simulink model "Simulacao_TCC_Final"  (Simulink 9.1)
settings: Solver=VariableStepAuto  StartTime=0.0  StopTime=11000  RelTol=1e-3
undefined symbols (not defined in the file or in its folder): magnitude
libraries: sharedutil x18, vrlib x5, simulink x2, aerolibanim x1
(part 1 of 2)
settings Model: Creator=Lucas  LastModifiedBy=Lucas
settings DataIOCC: SaveFormat=Dataset
settings OptimizationCC: LifeSpan=auto
settings DebuggingCC: UnderspecifiedInitializationDetection=Simplified  MergeDetectMultiDrivingBlocksExec=error  SFUnexpectedBacktrackingDiag=error  SFNoUnconditionalDefaultTransitionDiag=error  SFExecutionAtInitializationDiag=warning
settings HardwareCC: ProdBitPerPointer=64  ProdBitPerSizeT=64  ProdBitPerPtrDiffT=64  ProdLargestAtomicFloat=Float  ProdIntDivRoundTo=Zero  ProdEndianess=LittleEndian  ProdWordSize=64  ProdHWDeviceType=Intel->x86-64 (Windows64)
settings ModelReferenceCC: PropagateSignalLabelsOutOfModel=on
settings CodeAppCC: StateflowObjectComments=off
settings GRTTargetCC: TargetLangStandard=C99 (ISO)  CombineOutputUpdateFcns=on  GRTInterface=off
settings ConfigComp: CovMetricSettings=dwe  CovHtmlReporting=off  CovSaveCumulativeToWorkspaceVar=off  CovSaveSingleToWorkspaceVar=off  CovExternalEMLEnable=on

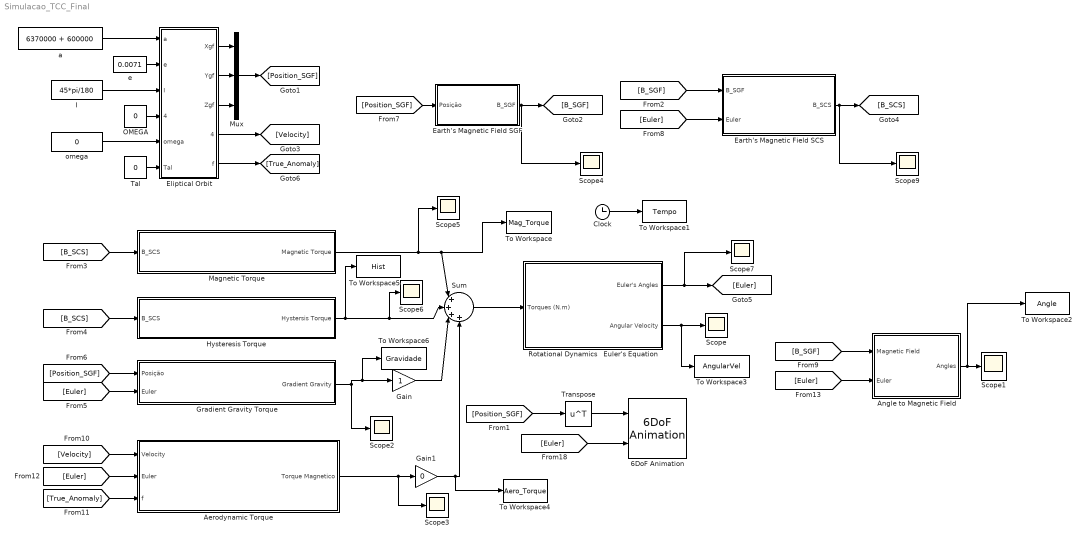
== system Simulacao_TCC_Final ==
  6DoF Animation : aerolibanim/6DoF Animation  u1=[-4000 4000 -2000 2000 -5000 -3000]  u2=10  u3=1000000*4  u4=[0 0 0]  u5=Fixed position  u6=[ 1 1 1 ] * 40000000  u7=15  u8=on
      settings: SourceProductName=Aerospace Blockset
  Aerodynamic Torque : Subsystem
  Angle to Magnetic Field : Subsystem
  Clock : Clock
  Earth's Magnetic Field SCS : Subsystem
  Earth's Magnetic Field SGF : Subsystem
  Eliptical Orbit : Subsystem
  Gain : Gain
  Gain1 : Gain  Gain=0
  Gradient Gravity Torque : Subsystem
  Hysteresis Torque : Subsystem
  I : Constant  Value=45*pi/180
  Magnetic Torque : Subsystem
  Mux : Mux  Inputs=3
  OMEGA : Constant  Value=0
  Rotational Dynamics   Euler's Equation : Subsystem
  Scope{,1..7,9} (9 alike) : Scope
  Sum : Sum  Inputs=|++++
  Tal : Constant  Value=0
  To Workspace : ToWorkspace  VariableName=Mag_Torque  SampleTime=-1
  To Workspace1 : ToWorkspace  VariableName=Tempo  SampleTime=-1
  To Workspace2 : ToWorkspace  VariableName=Angle  SampleTime=-1
  To Workspace3 : ToWorkspace  VariableName=AngularVel  SampleTime=-1
  To Workspace4 : ToWorkspace  VariableName=Aero_Torque  SampleTime=-1
  To Workspace5 : ToWorkspace  VariableName=Hist  SampleTime=-1
  To Workspace6 : ToWorkspace  VariableName=Gravidade  SampleTime=-1
  Transpose : Math  Operator=transpose  SaturateOnIntegerOverflow=on
  a : Constant  Value=6370000 + 600000
  e : Constant  Value=0.0071
  omega : Constant  Value=0
  wires:
  a/1 -> Eliptical Orbit/1(a)
  Eliptical Orbit/2(Ygf) -> Mux/2
  I/1 -> Eliptical Orbit/3(I)
  Tal/1 -> Eliptical Orbit/6(Tal)
  omega/1 -> Eliptical Orbit/5(omega)
  Eliptical Orbit/3(Zgf) -> Mux/3
  Eliptical Orbit/1(Xgf) -> Mux/1
  e/1 -> Eliptical Orbit/2(e)
  Mux/1 -> [Position_SGF]
  OMEGA/1 -> Eliptical Orbit/4(OMEGA)
  [Position_SGF] -> Earth's Magnetic Field SGF/1(Posição)
  Earth's Magnetic Field SGF/1(B_SGF) -> Scope4/1, [B_SGF]
  [B_SCS] -> Magnetic Torque/1(B_SCS)
  [B_SCS] -> Hysteresis Torque/1(B_SCS)
  [Euler] -> Gradient Gravity Torque/2(Euler)
  [Position_SGF] -> Gradient Gravity Torque/1(Posição)
  Sum/1 -> Rotational Dynamics   Euler's Equation/1(Torques (N.m))
  Magnetic Torque/1(Magnetic Torque) -> Scope5/1, To Workspace/1, Sum/1
  Hysteresis Torque/1(Hystersis Torque) -> Scope6/1, Sum/2, To Workspace5/1
  Rotational Dynamics   Euler's Equation/1(Euler's Angles) -> [Euler], Scope7/1
  [B_SGF] -> Angle to Magnetic Field/1(Magnetic Field)
  [Euler] -> Angle to Magnetic Field/2(Euler)
  Rotational Dynamics   Euler's Equation/2(Angular Velocity) -> To Workspace3/1, Scope/1
  Gradient Gravity Torque/1(Gradient Gravity) -> To Workspace6/1, Gain/1, Scope2/1
  Gain/1 -> Sum/3
  Earth's Magnetic Field SCS/1(B_SCS) -> Scope9/1, [B_SCS]
  [Euler] -> Earth's Magnetic Field SCS/2(Euler)
  [B_SGF] -> Earth's Magnetic Field SCS/1(B_SGF)
  [Euler] -> 6DoF Animation/2
  Transpose/1 -> 6DoF Animation/1
  [Position_SGF] -> Transpose/1
  Eliptical Orbit/4(Velocity) -> [Velocity]
  Eliptical Orbit/5(f) -> [True_Anomaly]
  Clock/1 -> To Workspace1/1
  Angle to Magnetic Field/1(Angles) -> To Workspace2/1, Scope1/1
  [Euler] -> Aerodynamic Torque/2(Euler)
  [True_Anomaly] -> Aerodynamic Torque/3(f)
  Aerodynamic Torque/1(Torque Magnetico) -> Scope3/1, Gain1/1
  Gain1/1 -> Sum/4, To Workspace4/1
  [Velocity] -> Aerodynamic Torque/1(Velocity)

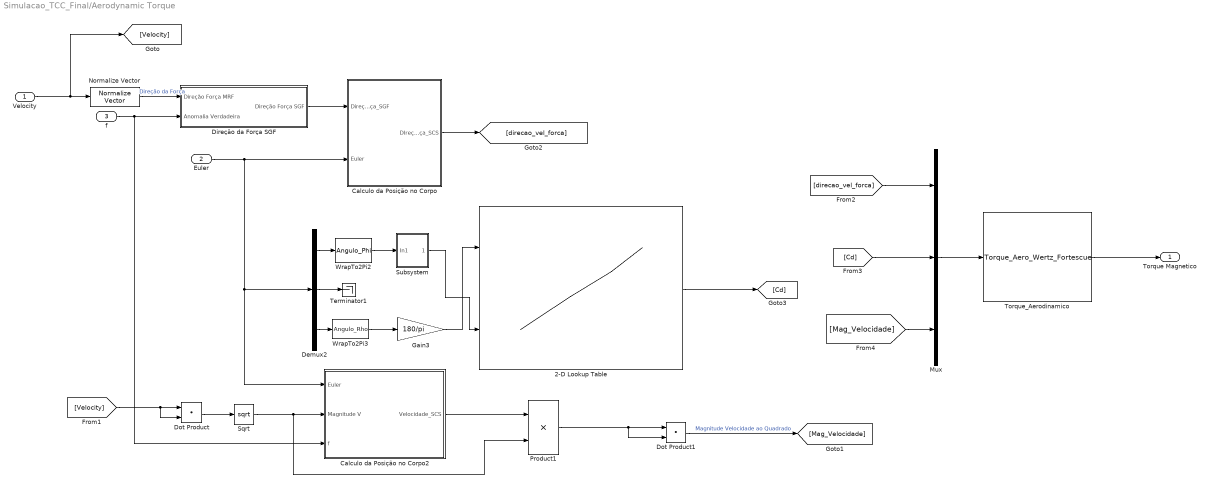
== system Simulacao_TCC_Final/Aerodynamic Torque ==
  Velocity : Inport
  Euler : Inport  Port=2
  f : Inport  Port=3
  2-D Lookup Table : Lookup_n-D  BreakpointsForDimension1=[0,45,90,135,180,225,270,315,360]  BreakpointsForDimension2=[0,10,20,30,40,50,60,70,80,90]  Table=reshape([2.7,1.93,2.7,1.93,2.7,1.93,2.7,1.93,2.47,2.7,1.9,2.47,1.9,2.7,1.9,2.47,1.9,2.45,2.7,1.85,2.25,1.85,2.7,1.85,2.25,1.85,2.43,2.7,1.83,2.07,1.83,2.7,1.83,2.07,1.83,2.41,2.7,1.8,1.95,1.8,2.7,1.8,1.95,1.8,2.39,2.7,1.8,1.95,1.8,2.7,1.8,1.95,1.8,2.39,2.7,1.83,2.07,1.83,2.7,1.83,2.07,1.83,2.41,2.7,1.85,2.25,1.85,2.7,1.85,2.25,1.85,2.43,2.7,1.9,2.47,1.9,2.7,1.9,2.47,1.9,2.47,2.7,1.93,2.7,1.93,2.7,1.93,2.7,1.93,2.47],9,10)  InternalRulePriority=Speed  RndMeth=Simplest  InputSameDT=on
  Calculo da Posição no Corpo : Subsystem
  Calculo da Posição no Corpo2 : Subsystem
  Demux2 : Demux  Outputs=3
  Direção da Força SGF : Subsystem
  Dot Product : DotProduct  InputSameDT=on  OutDataTypeStr=Inherit: Inherit via internal rule
  Dot Product1 : DotProduct  InputSameDT=on  OutDataTypeStr=Inherit: Inherit via internal rule
  Gain3 : Gain  Gain=180/pi
  Mux : Mux  Inputs=3
  Normalize Vector : vrlib/Utilities/Normalize Vector  maxzero=0
      settings: SourceProductName=Simulink 3D Animation  SourceProductBaseCode=VR
  Product1 : Product
  Sqrt : Sqrt  SaturateOnIntegerOverflow=on
  Subsystem : Subsystem
  Terminator1 : Terminator
  "Torque_Aerodinamico " : MATLABFcn  MATLABFcn=Torque_Aero_Wertz_Fortescue  OutputDimensions=3
  WrapTo2Pi2 : MATLABFcn  MATLABFcn=Angulo_Phi
  WrapTo2Pi3 : MATLABFcn  MATLABFcn=Angulo_Rho
  Torque Magnetico : Outport
  wires:
  Normalize Vector/1 -> Direção da Força SGF/1(Direção Força MRF)  "Direção da Força"
  Direção da Força SGF/1(Direção Força SGF) -> Calculo da Posição no Corpo/1(Direção_Força_SGF)
  Calculo da Posição no Corpo/1(DIreção_Força_SCS) -> [direcao_vel_forca]
  Velocity/1 -> [Velocity], Normalize Vector/1
  f/1 -> Calculo da Posição no Corpo2/3(f), Direção da Força SGF/2(Anomalia Verdadeira)
  Calculo da Posição no Corpo2/1("Velocidade_SCS ") -> Product1/1
  Dot Product/1 -> Sqrt/1
  [Velocity] -> Dot Product/2, Dot Product/1
  Euler/1 -> Demux2/1, Calculo da Posição no Corpo2/1(Euler), Calculo da Posição no Corpo/2(Euler)
  Dot Product1/1 -> [Mag_Velocidade]  "Magnitude Velocidade ao Quadrado"
  [direcao_vel_forca] -> Mux/1
  [Cd] -> Mux/2
  [Mag_Velocidade] -> Mux/3
  Mux/1 -> "Torque_Aerodinamico "/1
  "Torque_Aerodinamico "/1 -> Torque Magnetico/1
  Sqrt/1 -> Product1/2, Calculo da Posição no Corpo2/2(Magnitude V)
  Product1/1 -> Dot Product1/2, Dot Product1/1
  Demux2/2 -> Terminator1/1
  Subsystem/1(Out1) -> 2-D Lookup Table/2
  WrapTo2Pi2/1 -> Subsystem/1(In1)
  2-D Lookup Table/1 -> [Cd]
  Demux2/3 -> WrapTo2Pi3/1
  Gain3/1 -> 2-D Lookup Table/1
  Demux2/1 -> WrapTo2Pi2/1
  WrapTo2Pi3/1 -> Gain3/1

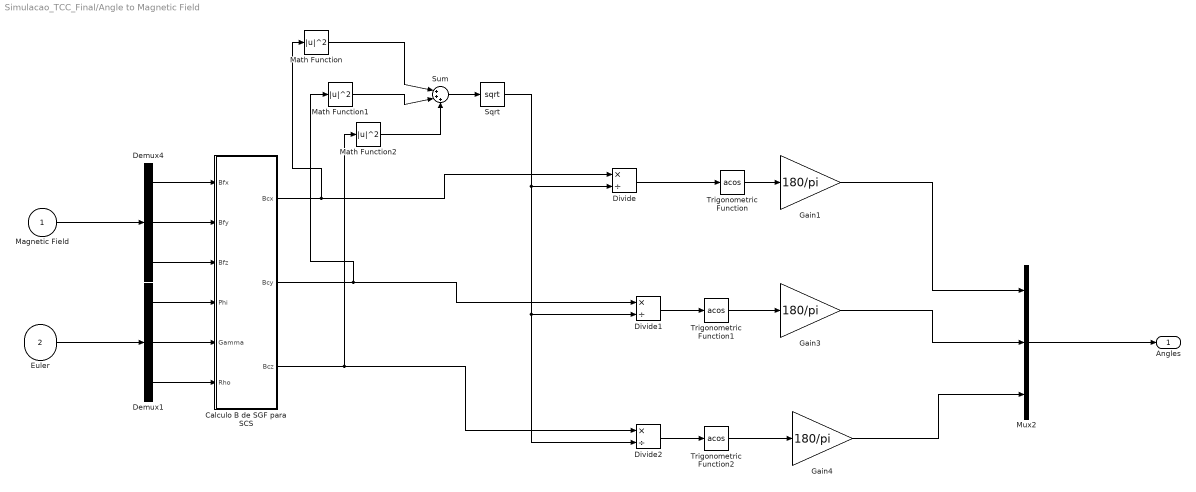
== system Simulacao_TCC_Final/Angle to Magnetic Field ==
  Magnetic Field : Inport
  Euler : Inport  Port=2
  Calculo B de SGF para SCS : Subsystem
  Demux1 : Demux  Outputs=3
  Demux4 : Demux  Outputs=3
  Divide : Product  Inputs=*/
  Divide1 : Product  Inputs=*/
  Divide2 : Product  Inputs=*/
  Gain1 : Gain  Gain=180/pi
  Gain3 : Gain  Gain=180/pi
  Gain4 : Gain  Gain=180/pi
  Math Function : Math  Operator=magnitude^2  SaturateOnIntegerOverflow=on
  Math Function1 : Math  Operator=magnitude^2  SaturateOnIntegerOverflow=on
  Math Function2 : Math  Operator=magnitude^2  SaturateOnIntegerOverflow=on
  Mux2 : Mux  Inputs=3
  Sqrt : Sqrt  SaturateOnIntegerOverflow=on
  Sum : Sum  Inputs=|+++
  Trigonometric Function : Trigonometry  Operator=acos
  Trigonometric Function1 : Trigonometry  Operator=acos
  Trigonometric Function2 : Trigonometry  Operator=acos
  Angles : Outport
  wires:
  Demux4/1 -> Calculo B de SGF para SCS/1(Bfx)
  Demux4/2 -> Calculo B de SGF para SCS/2(Bfy)
  Demux4/3 -> Calculo B de SGF para SCS/3(Bfz)
  Magnetic Field/1 -> Demux4/1
  Demux1/1 -> Calculo B de SGF para SCS/4(Phi)
  Demux1/2 -> Calculo B de SGF para SCS/5(Gamma)
  Demux1/3 -> Calculo B de SGF para SCS/6(Rho)
  Euler/1 -> Demux1/1
  Mux2/1 -> Angles/1
  Trigonometric Function2/1 -> Gain4/1
  Trigonometric Function1/1 -> Gain3/1
  Divide1/1 -> Trigonometric Function1/1
  Divide2/1 -> Trigonometric Function2/1
  Trigonometric Function/1 -> Gain1/1
  Divide/1 -> Trigonometric Function/1
  Calculo B de SGF para SCS/1(Bcx) -> Math Function/1, Divide/1
  Sqrt/1 -> Divide2/2, Divide1/2, Divide/2
  Calculo B de SGF para SCS/2(Bcy) -> Math Function1/1, Divide1/1
  Calculo B de SGF para SCS/3(Bcz) -> Divide2/1, Math Function2/1
  Gain1/1 -> Mux2/1
  Gain3/1 -> Mux2/2
  Gain4/1 -> Mux2/3
  Sum/1 -> Sqrt/1
  Math Function/1 -> Sum/1
  Math Function1/1 -> Sum/2
  Math Function2/1 -> Sum/3

== system Simulacao_TCC_Final/Earth's Magnetic Field SCS ==
  B_SGF : Inport
  Euler : Inport  Port=2
  Demux2 : Demux  Outputs=3
  Matrix Multiply : Product  Multiplication=Matrix(*)
  Matrix Multiply1 : Product  Multiplication=Matrix(*)
  Matrix Multiply2 : Product  Multiplication=Matrix(*)
  Matrix de Rotação em X : Subsystem
  Matrix de Rotação em Y : Subsystem
  Matrix de Rotação em Z : Subsystem
  B_SCS : Outport
  wires:
  Euler/1 -> Demux2/1
  Matrix Multiply/1 -> B_SCS/1
  B_SGF/1 -> Matrix Multiply/2
  Demux2/1 -> Matrix de Rotação em X/1(Phi)
  Demux2/2 -> Matrix de Rotação em Y/1(Gamma)
  Demux2/3 -> Matrix de Rotação em Z/1(Phi)
  Matrix de Rotação em X/1(Matrix Rotação  em X) -> Matrix Multiply1/1
  Matrix de Rotação em Y/1(Matrix Rotação  em Y) -> Matrix Multiply1/2
  Matrix Multiply1/1 -> Matrix Multiply2/1
  Matrix de Rotação em Z/1(Matrix Rotação  em Z) -> Matrix Multiply2/2
  Matrix Multiply2/1 -> Matrix Multiply/1

== system Simulacao_TCC_Final/Earth's Magnetic Field SGF ==
  Posição : Inport
  1 : Math  Operator=magnitude^2  SaturateOnIntegerOverflow=on
  2 : Math  Operator=magnitude^2  SaturateOnIntegerOverflow=on
  3 : Math  Operator=magnitude^2  SaturateOnIntegerOverflow=on
  Calculo Campo Magnetico LATITUDE : Subsystem
  Demux : Demux  Outputs=3
  Demux1 : Demux  Outputs=3
  Mux2 : Mux  Inputs=3
  Raio Terra : Constant  Value=6370000
  SGF para SGG : Subsystem
  SGF para SGG1 : Subsystem
  SGF para SGG2 : Subsystem
  SGF para SGG3 : Subsystem
  Sist Esferico - > SMG1 : Subsystem
  Sqrt : Sqrt  SaturateOnIntegerOverflow=on
  Sum : Sum  Inputs=|+++
  B_SGF : Outport
  wires:
  Demux/1 -> 1/1
  Demux/2 -> 2/1
  Raio Terra/1 -> Calculo Campo Magnetico LATITUDE/2(Raio Terra)
  Sum/1 -> Sqrt/1
  1/1 -> Sum/1
  2/1 -> Sum/2
  3/1 -> Sum/3
  Demux/3 -> 3/1
  Posição/1 -> SGF para SGG/1(Posição_SGF), Demux/1
  Sqrt/1 -> [Raio]  "RAIO"
  SGF para SGG/1(Posição_SGG) -> SGF para SGG1/1(Posição_SGG)
  SGF para SGG1/1(Posição_SMG) -> Demux1/1
  Demux1/3 -> Calculo Campo Magnetico LATITUDE/1(Zgm), Sist Esferico - > SMG1/6(Zm)
  [Raio] -> Calculo Campo Magnetico LATITUDE/3(Raio)
  Calculo Campo Magnetico LATITUDE/1(Br) -> Sist Esferico - > SMG1/1(Br)
  Calculo Campo Magnetico LATITUDE/2(Btheta) -> Sist Esferico - > SMG1/2(Btheta)
  Calculo Campo Magnetico LATITUDE/3(Delta) -> Sist Esferico - > SMG1/3(Delta)
  Demux1/1 -> Sist Esferico - > SMG1/4(Xm)
  Demux1/2 -> Sist Esferico - > SMG1/5(Ym)
  Mux2/1 -> SGF para SGG2/1(B_SMG)
  Sist Esferico - > SMG1/1(Bmx) -> Mux2/1
  Sist Esferico - > SMG1/2(Bmy) -> Mux2/2
  Sist Esferico - > SMG1/3(Bmz) -> Mux2/3
  SGF para SGG2/1(B_SGG) -> SGF para SGG3/1(B_SGG)
  SGF para SGG3/1(B_SGF) -> B_SGF/1

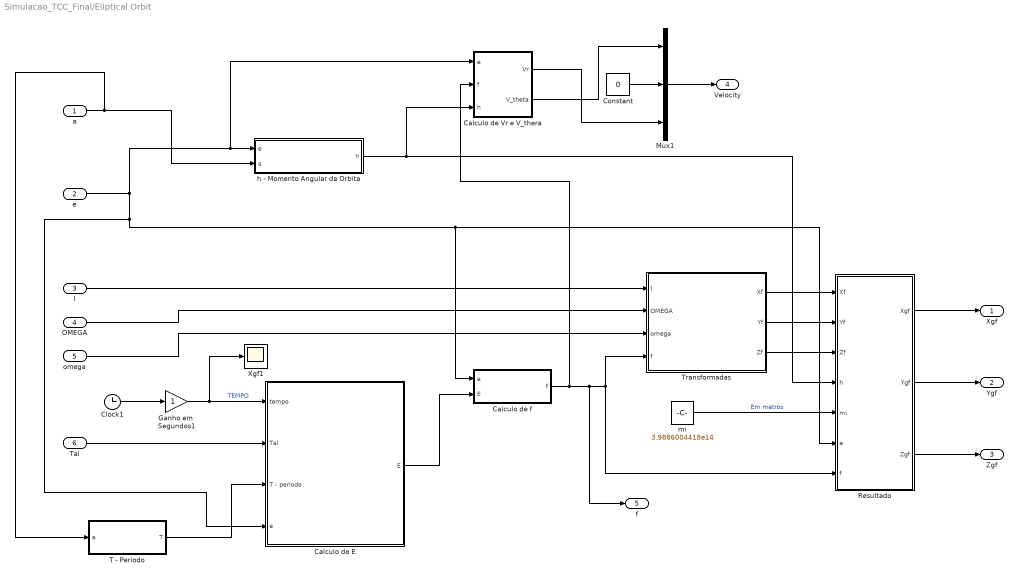
== system Simulacao_TCC_Final/Eliptical Orbit ==
  a : Inport
  e : Inport  Port=2
  I : Inport  Port=3
  OMEGA : Inport  Port=4
  omega : Inport  Port=5
  Tal : Inport  Port=6
  Calculo de E : Subsystem
  Calculo de Vr e V_thera : Subsystem
  Calculo de f : Subsystem
  Clock1 : Clock
  Constant : Constant  Value=0
  Ganho em  Segundos1 : Gain
  Mux1 : Mux  Inputs=3
  Resultado : Subsystem
  T - Periodo : Subsystem
  Transformadas : Subsystem
  Xgf1 : Scope
  h - Momento Angular da Orbita : Subsystem
  mi : Constant  Value=3.9886004418e14
  Xgf : Outport
  Ygf : Outport  Port=2
  Zgf : Outport  Port=3
  Velocity : Outport  Port=4
  f : Outport  Port=5
  wires:
  Transformadas/2(Yf) -> Resultado/2(Yf)
  Transformadas/3(Zf) -> Resultado/3(Zf)
  Calculo de f/1(f) -> Calculo de Vr e V_thera/2(f), f/1, Transformadas/4(f), Resultado/7(f)
  Transformadas/1(Xf) -> Resultado/1(Xf)
  mi/1 -> Resultado/5(mi)  "Em metros"
  e/1 -> Calculo de E/4("e  "), Calculo de f/1(e), Resultado/6(e), Calculo de Vr e V_thera/1(e), h - Momento Angular da Orbita/1(e)
  h - Momento Angular da Orbita/1(h) -> Calculo de Vr e V_thera/3(h), Resultado/4(h)
  I/1 -> Transformadas/1(I)
  OMEGA/1 -> Transformadas/2(OMEGA)
  omega/1 -> Transformadas/3(omega)
  Resultado/3(Zgf) -> Zgf/1
  Resultado/2(Ygf) -> Ygf/1
  Resultado/1(Xgf) -> Xgf/1
  Tal/1 -> Calculo de E/2(Tal)
  T - Periodo/1(T) -> Calculo de E/3(T - periodo)
  a/1 -> T - Periodo/1(a), h - Momento Angular da Orbita/2(a)
  Clock1/1 -> Ganho em  Segundos1/1
  Ganho em  Segundos1/1 -> Xgf1/1, Calculo de E/1(tempo)  "TEMPO"
  Calculo de E/1(E) -> Calculo de f/2(E)
  Calculo de Vr e V_thera/1(Vr) -> Mux1/3
  Constant/1 -> Mux1/2
  Calculo de Vr e V_thera/2(V_theta) -> Mux1/1
  Mux1/1 -> Velocity/1

== system Simulacao_TCC_Final/Gradient Gravity Torque ==
  note: Vetor Nadir
  Posição : Inport
  Euler : Inport  Port=2
  3u. : Gain  Gain=3*(3.9886004418e14)
  Calculo da Posição no Corpo : Subsystem
  Constant : Constant  Value=0
  Cross Product : vrlib/Utilities/Cross Product
      settings: SourceProductBaseCode=VR
  Divide : Product  Inputs=*/
  Dot Product : DotProduct  InputSameDT=on  OutDataTypeStr=Inherit: Inherit via internal rule
  Gain : Gain  Gain=-1
  Gain1 : Gain  Gain=-1
  Ixx : Constant  Value=0.00182
  Iyy : Constant  Value=0.00185
  Izz : Constant  Value=0.00220
  Math Function : Math  Operator=square  SaturateOnIntegerOverflow=on
  Matrix Multiply : Product  Multiplication=Matrix(*)
  Matriz de Inercia : sharedutil/Create 3x3 Matrix  aMode=aMode
  Normalize Vector : vrlib/Utilities/Normalize Vector  maxzero=0
      settings: SourceProductName=Simulink 3D Animation  SourceProductBaseCode=VR
  Gradient Gravity : Outport
  wires:
  Euler/1 -> Calculo da Posição no Corpo/2(Euler)
  Calculo da Posição no Corpo/1(X_SCS) -> Gain1/1, Normalize Vector/1
  Normalize Vector/1 -> Gain/1
  Gain/1 -> Matrix Multiply/2
  Posição/1 -> Dot Product/2, Dot Product/1, Calculo da Posição no Corpo/1(X_SGF)
  Constant/1 -> Matriz de Inercia/4, Matriz de Inercia/3, Matriz de Inercia/2, Matriz de Inercia/6, Matriz de Inercia/7, Matriz de Inercia/8
  Ixx/1 -> Matriz de Inercia/1
  Iyy/1 -> Matriz de Inercia/5
  Izz/1 -> Matriz de Inercia/9
  Matriz de Inercia/1 -> Matrix Multiply/1
  Divide/1 -> Cross Product/1
  Matrix Multiply/1 -> Cross Product/2
  Cross Product/1 -> Gradient Gravity/1
  Dot Product/1 -> Math Function/1
  Math Function/1 -> Divide/2
  3u./1 -> Divide/1
  Gain1/1 -> 3u./1

== system Simulacao_TCC_Final/Hysteresis Torque ==
  B_SCS : Inport
  1/mu : Gain  Gain=1/(1.256637061435917e-06)
  1/mu. : Constant  Value=1/(1.256637061435917e-06)
  Cross Product : vrlib/Utilities/Cross Product
      settings: SourceProductBaseCode=VR
  Hysteresys : Subsystem
  V/mu : Product  RndMeth=Zero
  Volume Material : Constant  Value=[5e-9 7e-08 7e-08]
  m : Product  RndMeth=Zero
  Hystersis Torque : Outport
  wires:
  B_SCS/1 -> 1/mu/1, Cross Product/2
  m/1 -> Cross Product/1
  Hysteresys/1(B) -> m/1
  1/mu/1 -> Hysteresys/1(H)
  Cross Product/1 -> Hystersis Torque/1
  Volume Material/1 -> V/mu/1
  1/mu./1 -> V/mu/2
  V/mu/1 -> m/2

== system Simulacao_TCC_Final/Magnetic Torque ==
  note: T = m X B
  B_SCS : Inport
  Cross Product : vrlib/Utilities/Cross Product
      settings: SourceProductBaseCode=VR
  Imãs : Constant  Value=[0.7 0 0]
  Magnetic Torque : Outport
  wires:
  B_SCS/1 -> Cross Product/2  "Magnetic Field on Body"
  Imãs/1 -> Cross Product/1
  Cross Product/1 -> Magnetic Torque/1

== system Simulacao_TCC_Final/Rotational Dynamics   Euler's Equation ==
  Torques (N.m) : Inport
  Euler Angles : Subsystem
  Euler's Equation Body - Framed : Subsystem
  Euler's Angles : Outport
  Angular Velocity : Outport  Port=2
  wires:
  Torques (N.m)/1 -> Euler's Equation Body - Framed/1(Torques)
  Euler's Equation Body - Framed/1(Angular Velocity Body Frame) -> Angular Velocity/1, Euler Angles/1(Angular Velocity Body Frame)
  Euler Angles/1(Euler's Angle) -> Euler's Angles/1

== system Simulacao_TCC_Final/Aerodynamic Torque/Calculo da Posição no Corpo ==
  Direção_Força_SGF : Inport
  Euler : Inport  Port=2
  Demux1 : Demux  Outputs=3
  Matrix Multiply : Product  Multiplication=Matrix(*)
  Matrix Multiply1 : Product  Multiplication=Matrix(*)
  Matrix Multiply2 : Product  Multiplication=Matrix(*)
  Matrix de Rotação em X : Subsystem
  Matrix de Rotação em Y : Subsystem
  Matrix de Rotação em Z : Subsystem
  DIreção_Força_SCS : Outport
  wires:
  Direção_Força_SGF/1 -> Matrix Multiply/2
  Matrix Multiply/1 -> DIreção_Força_SCS/1
  Matrix de Rotação em X/1(Matrix Rotação  em X) -> Matrix Multiply1/1
  Euler/1 -> Demux1/1
  Demux1/3 -> Matrix de Rotação em Z/1(Phi)
  Matrix de Rotação em Z/1(Matrix Rotação  em Z) -> Matrix Multiply2/2
  Matrix de Rotação em Y/1(Matrix Rotação  em Y) -> Matrix Multiply1/2
  Demux1/2 -> Matrix de Rotação em Y/1(Gamma)
  Matrix Multiply1/1 -> Matrix Multiply2/1
  Matrix Multiply2/1 -> Matrix Multiply/1
  Demux1/1 -> Matrix de Rotação em X/1(Phi)

== system Simulacao_TCC_Final/Aerodynamic Torque/Calculo da Posição no Corpo2 ==
  Euler : Inport
  Magnitude V : Inport  Port=2
  f : Inport  Port=3
  Constant : Constant  Value=-1
  Constant1 : Constant  Value=6370000 + 300000
  Constant2 : Constant  Value=0
  Constant3 : Constant  Value=7.27e-5
  Demux1 : Demux  Outputs=3
  Divide : Product  Inputs=*/
  Matrix Multiply : Product  Multiplication=Matrix(*)
  Matrix Multiply1 : Product  Multiplication=Matrix(*)
  Matrix Multiply2 : Product  Multiplication=Matrix(*)
  Matrix de Rotação em X : Subsystem
  Matrix de Rotação em Y : Subsystem
  Matrix de Rotação em Z : Subsystem
  Mux : Mux  Inputs=3
  Product : Product  Inputs=3
  Trigonometric Function : Trigonometry  Operator=cos
  "Velocidade_SCS " : Outport
  wires:
  Matrix Multiply/1 -> "Velocidade_SCS "/1
  Matrix de Rotação em X/1(Matrix Rotação  em X) -> Matrix Multiply1/1
  Euler/1 -> Demux1/1
  Demux1/3 -> Matrix de Rotação em Z/1(Phi)
  Matrix de Rotação em Z/1(Matrix Rotação  em Z) -> Matrix Multiply2/2
  Matrix de Rotação em Y/1(Matrix Rotação  em Y) -> Matrix Multiply1/2
  Demux1/2 -> Matrix de Rotação em Y/1(Gamma)
  Matrix Multiply1/1 -> Matrix Multiply2/1
  Matrix Multiply2/1 -> Matrix Multiply/1
  Demux1/1 -> Matrix de Rotação em X/1(Phi)
  Mux/1 -> Matrix Multiply/2
  Constant/1 -> Mux/1
  Divide/1 -> Product/2
  Magnitude V/1 -> Divide/2
  Constant1/1 -> Divide/1
  f/1 -> Trigonometric Function/1
  Trigonometric Function/1 -> Product/1
  Constant2/1 -> Mux/3
  Product/1 -> Mux/2
  Constant3/1 -> Product/3

== system Simulacao_TCC_Final/Aerodynamic Torque/Direção da Força SGF ==
  Direção Força MRF : Inport
  Anomalia Verdadeira : Inport  Port=2
  Add : Sum
  Constant : Constant  Value=pi/2
  Constant1 : Constant  Value=0
  Demux : Demux  Outputs=3
  Mux1 : Mux  Inputs=3
  Product : Product
  Product1 : Product
  Terminator1 : Terminator
  Terminator2 : Terminator
  Trigonometric Function : Trigonometry  Operator=cos
  Trigonometric Function1 : Trigonometry
  Direção Força SGF : Outport
  wires:
  Mux1/1 -> Direção Força SGF/1
  Constant/1 -> Add/1
  Anomalia Verdadeira/1 -> Add/2
  Add/1 -> Trigonometric Function1/1, Trigonometric Function/1
  Direção Força MRF/1 -> Demux/1
  Product1/1 -> Mux1/2
  Trigonometric Function/1 -> Product/1
  Trigonometric Function1/1 -> Product1/1
  Demux/1 -> Product1/2, Product/2
  Product/1 -> Mux1/1
  Constant1/1 -> Mux1/3
  Demux/3 -> Terminator2/1
  Demux/2 -> Terminator1/1

== system Simulacao_TCC_Final/Aerodynamic Torque/Subsystem ==
  In1 : Inport
  Gain1 : Gain  Gain=180/pi
  If : If  IfExpression=u1 > 90
  If Action Subsystem1 : Subsystem  TreatAsAtomicUnit=on
  If Action Subsystem2 : Subsystem  TreatAsAtomicUnit=on
  Merge : Merge
  Out1 : Outport
  wires:
  In1/1 -> Gain1/1
  Gain1/1 -> [A], If/1
  Merge/1 -> Out1/1
  If/1 -> If Action Subsystem1/Action
  [A] -> If Action Subsystem1/1(In1)
  If/2 -> If Action Subsystem2/Action
  [A] -> If Action Subsystem2/1(In1)
  If Action Subsystem2/1(Out1) -> Merge/2
  If Action Subsystem1/1(Out1) -> Merge/1

== system Simulacao_TCC_Final/Angle to Magnetic Field/Calculo B de SGF para SCS ==
  Bfx : Inport
  Bfy : Inport  Port=2
  Bfz : Inport  Port=3
  Phi : Inport  Port=4
  Gamma : Inport  Port=5
  Rho : Inport  Port=6
  "Calculo de X " : Subsystem
  Calculo de Y : Subsystem
  Calculo de Z : Subsystem
  Gain : Gain
  Bcx : Outport
  Bcy : Outport  Port=2
  Bcz : Outport  Port=3
  wires:
  Bfz/1 -> Calculo de Z/3(Bfz), Calculo de Y/3(Bfz), "Calculo de X "/3(Bfz)
  "Calculo de X "/1(X) -> Gain/1
  Calculo de Y/1(Y) -> Bcy/1
  Calculo de Z/1(Z) -> Bcz/1
  Bfx/1 -> Calculo de Z/1(Bfx), Calculo de Y/1(Bfx), "Calculo de X "/1(Bfx)
  Bfy/1 -> Calculo de Z/2(Bfy), Calculo de Y/2(Bfy), "Calculo de X "/2(Bfy)
  Phi/1 -> Calculo de Z/4(Phi), Calculo de Y/4(Phi)
  Gamma/1 -> "Calculo de X "/4(Gamma), Calculo de Z/5(Gamma), Calculo de Y/5(Gamma)
  Rho/1 -> "Calculo de X "/5(Rho), Calculo de Z/6(Rho), Calculo de Y/6(Rho)
  Gain/1 -> Bcx/1

== system Simulacao_TCC_Final/Earth's Magnetic Field SCS/Matrix de Rotação em X ==
  Phi : Inport
  Constant : Constant
  Constant{1..4} (4 alike) : Constant  Value=0
  Create 3x3 Matrix : sharedutil/Create 3x3 Matrix  aMode=aMode
  Gain : Gain  Gain=-1
  Trigonometric Function : Trigonometry
  Trigonometric Function1 : Trigonometry  Operator=cos
  Trigonometric Function2 : Trigonometry
  Trigonometric Function3 : Trigonometry  Operator=cos
  Matrix Rotação  em X : Outport
  wires:
  Constant/1 -> Create 3x3 Matrix/1
  Constant1/1 -> Create 3x3 Matrix/2
  Constant2/1 -> Create 3x3 Matrix/3
  Constant3/1 -> Create 3x3 Matrix/4
  Trigonometric Function1/1 -> Create 3x3 Matrix/5
  Trigonometric Function/1 -> Create 3x3 Matrix/6
  Constant4/1 -> Create 3x3 Matrix/7
  Phi/1 -> Trigonometric Function2/1, Trigonometric Function3/1, Trigonometric Function/1, Trigonometric Function1/1
  Trigonometric Function2/1 -> Gain/1
  Gain/1 -> Create 3x3 Matrix/8
  Trigonometric Function3/1 -> Create 3x3 Matrix/9
  Create 3x3 Matrix/1 -> Matrix Rotação  em X/1

== system Simulacao_TCC_Final/Earth's Magnetic Field SCS/Matrix de Rotação em Y ==
  Gamma : Inport
  Constant : Constant
  Constant{1..4} (4 alike) : Constant  Value=0
  Create 3x3 Matrix : sharedutil/Create 3x3 Matrix  aMode=aMode
  Gain : Gain  Gain=-1
  Trigonometric Function : Trigonometry
  Trigonometric Function1 : Trigonometry  Operator=cos
  Trigonometric Function2 : Trigonometry
  Trigonometric Function3 : Trigonometry  Operator=cos
  Matrix Rotação  em Y : Outport
  wires:
  Create 3x3 Matrix/1 -> Matrix Rotação  em Y/1
  Trigonometric Function1/1 -> Create 3x3 Matrix/1
  Trigonometric Function2/1 -> Gain/1
  Constant1/1 -> Create 3x3 Matrix/2
  Gain/1 -> Create 3x3 Matrix/3
  Constant2/1 -> Create 3x3 Matrix/4
  Constant/1 -> Create 3x3 Matrix/5
  Constant3/1 -> Create 3x3 Matrix/6
  Trigonometric Function/1 -> Create 3x3 Matrix/7
  Constant4/1 -> Create 3x3 Matrix/8
  Trigonometric Function3/1 -> Create 3x3 Matrix/9
  Gamma/1 -> Trigonometric Function/1, Trigonometric Function3/1, Trigonometric Function1/1, Trigonometric Function2/1

== system Simulacao_TCC_Final/Earth's Magnetic Field SCS/Matrix de Rotação em Z ==
  Phi : Inport
  Constant : Constant
  Constant{1..4} (4 alike) : Constant  Value=0
  Create 3x3 Matrix : sharedutil/Create 3x3 Matrix  aMode=aMode
  Gain : Gain  Gain=-1
  Trigonometric Function : Trigonometry
  Trigonometric Function1 : Trigonometry  Operator=cos
  Trigonometric Function2 : Trigonometry
  Trigonometric Function3 : Trigonometry  Operator=cos
  Matrix Rotação  em Z : Outport
  wires:
  Create 3x3 Matrix/1 -> Matrix Rotação  em Z/1
  Trigonometric Function2/1 -> Gain/1
  Trigonometric Function1/1 -> Create 3x3 Matrix/1
  Trigonometric Function/1 -> Create 3x3 Matrix/2
  Constant2/1 -> Create 3x3 Matrix/3
  Gain/1 -> Create 3x3 Matrix/4
  Trigonometric Function3/1 -> Create 3x3 Matrix/5
  Constant3/1 -> Create 3x3 Matrix/6
  Constant1/1 -> Create 3x3 Matrix/7
  Constant4/1 -> Create 3x3 Matrix/8
  Constant/1 -> Create 3x3 Matrix/9
  Phi/1 -> Trigonometric Function/1, Trigonometric Function1/1, Trigonometric Function2/1, Trigonometric Function3/1

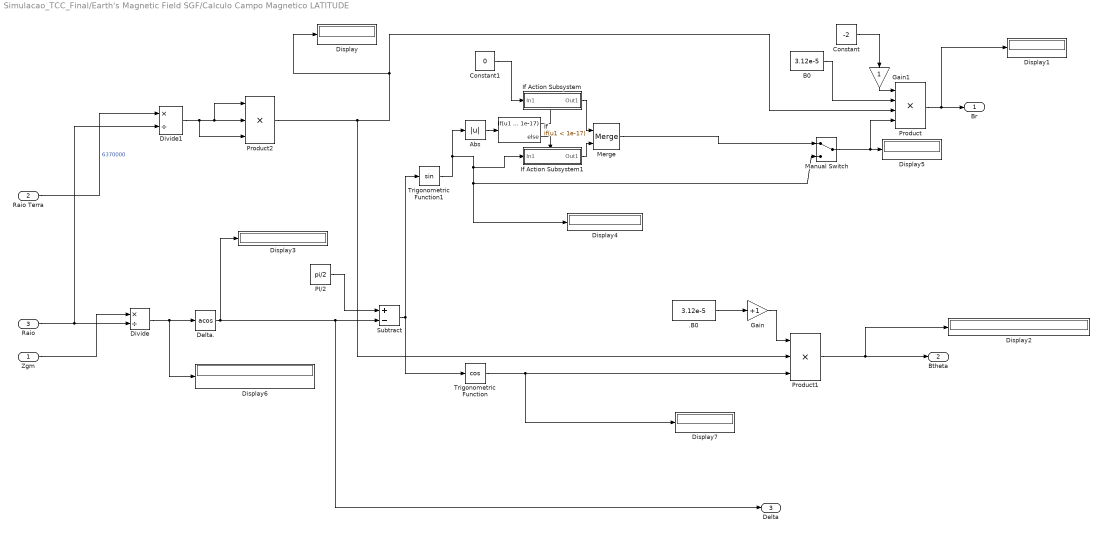
== system Simulacao_TCC_Final/Earth's Magnetic Field SGF/Calculo Campo Magnetico LATITUDE ==
  Zgm : Inport
  Raio Terra : Inport  Port=2
  Raio : Inport  Port=3
  .B0 : Constant  Value=3.12e-5
  Abs : Abs
  B0 : Constant  Value=3.12e-5
  Constant : Constant  Value=-2
  Constant1 : Constant  Value=0
  Delta. : Trigonometry  Operator=acos  OutputSignalType=real
  Display{,1..7} (8 alike) : Display
  Divide : Product  Inputs=*/
  Divide1 : Product  Inputs=*/
  Gain : Gain  Gain=+1
  Gain1 : Gain
  If : If  IfExpression=u1 < 1e-17
  If Action Subsystem : Subsystem  TreatAsAtomicUnit=on
  If Action Subsystem1 : Subsystem  TreatAsAtomicUnit=on
  Manual Switch : ManualSwitch
  Merge : Merge
  "PI/2 " : Constant  Value=pi/2
  Product : Product  Inputs=4
  Product1 : Product  Inputs=3
  Product2 : Product  Inputs=3
  Subtract : Sum  Inputs=+-
  Trigonometric Function : Trigonometry  Operator=cos
  Trigonometric Function1 : Trigonometry  ApproximationMethod=CORDIC  NumberOfIterations=100
  Br : Outport
  Btheta : Outport  Port=2
  Delta : Outport  Port=3
  wires:
  Zgm/1 -> Divide/1
  Raio/1 -> Divide1/2, Divide/2
  Divide/1 -> Display6/1, Delta./1
  Trigonometric Function1/1 -> Abs/1, If Action Subsystem1/1(In1), Display4/1, Manual Switch/2
  Constant/1 -> Gain1/1
  B0/1 -> Product/2
  Raio Terra/1 -> Divide1/1  "6370000"
  Product/1 -> Display1/1, Br/1
  Product2/1 -> Display/1, Product/3, Product1/2
  Product1/1 -> Display2/1, Btheta/1
  .B0/1 -> Gain/1
  Divide1/1 -> Product2/3, Product2/1, Product2/2
  Manual Switch/1 -> Product/4, Display5/1
  Merge/1 -> Manual Switch/1
  If Action Subsystem/1(Out1) -> Merge/1
  If Action Subsystem1/1(Out1) -> Merge/2
  If/1 -> If Action Subsystem/Action
  If/2 -> If Action Subsystem1/Action
  Constant1/1 -> If Action Subsystem/1(In1)
  Abs/1 -> If/1
  Gain/1 -> Product1/1
  Trigonometric Function/1 -> Display7/1, Product1/3
  Gain1/1 -> Product/1
  "PI/2 "/1 -> Subtract/1
  Delta./1 -> Subtract/2, Delta/1, Display3/1
  Subtract/1 -> Trigonometric Function/1, Trigonometric Function1/1

== system Simulacao_TCC_Final/Earth's Magnetic Field SGF/SGF para SGG ==
  Posição_SGF : Inport
  Constant{1..4} (4 alike) : Constant  Value=0
  Constant5 : Constant
  Gain : Gain
  Gain1 : Gain  Gain=-1
  Matriz Rotação ao Redor de Z Antihorária : sharedutil/Create 3x3 Matrix  aMode=aMode
  Rotação da Terra : simulink/Sources/Ramp  slope="7.292115856e-5   %2*pi/(24*60*60)  %radians/second (one rotation per day )"  start=0  InitialOutput=0
  Trigonometric Function : Trigonometry
  Trigonometric Function1 : Trigonometry  Operator=cos
  Trigonometric Function2 : Trigonometry
  Trigonometric Function3 : Trigonometry  Operator=cos
  product 2 : Product  Multiplication=Matrix(*)  RndMeth=Zero
  Posição_SGG : Outport
  wires:
  Rotação da Terra/1 -> Gain/1
  product 2/1 -> Posição_SGG/1
  Trigonometric Function1/1 -> Matriz Rotação ao Redor de Z Antihorária/1
  Trigonometric Function/1 -> Gain1/1
  Gain1/1 -> Matriz Rotação ao Redor de Z Antihorária/2
  Constant1/1 -> Matriz Rotação ao Redor de Z Antihorária/3
  Trigonometric Function2/1 -> Matriz Rotação ao Redor de Z Antihorária/4
  Trigonometric Function3/1 -> Matriz Rotação ao Redor de Z Antihorária/5
  Constant2/1 -> Matriz Rotação ao Redor de Z Antihorária/6
  Constant3/1 -> Matriz Rotação ao Redor de Z Antihorária/7
  Constant4/1 -> Matriz Rotação ao Redor de Z Antihorária/8
  Constant5/1 -> Matriz Rotação ao Redor de Z Antihorária/9
  Matriz Rotação ao Redor de Z Antihorária/1 -> product 2/1  "Matriz de Rotação"
  Posição_SGF/1 -> product 2/2
  Gain/1 -> Trigonometric Function2/1, Trigonometric Function3/1, Trigonometric Function/1, Trigonometric Function1/1

== system Simulacao_TCC_Final/Earth's Magnetic Field SGF/SGF para SGG1 ==
  Posição_SGG : Inport
  Constant{1..4} (4 alike) : Constant  Value=0
  Constant5 : Constant
  Constant6 : Constant  Value=11*(pi/180)
  Gain : Gain
  Gain1 : Gain  Gain=-1
  Matriz Rotação ao Redor de Z Antihorária : sharedutil/Create 3x3 Matrix  aMode=aMode
  Trigonometric Function : Trigonometry
  Trigonometric Function1 : Trigonometry  Operator=cos
  Trigonometric Function2 : Trigonometry
  Trigonometric Function3 : Trigonometry  Operator=cos
  product 2 : Product  Multiplication=Matrix(*)  RndMeth=Zero
  Posição_SMG : Outport
  wires:
  Constant6/1 -> Gain/1
  product 2/1 -> Posição_SMG/1
  Trigonometric Function/1 -> Gain1/1
  Matriz Rotação ao Redor de Z Antihorária/1 -> product 2/1  "Matriz de Rotação"
  Posição_SGG/1 -> product 2/2
  Constant5/1 -> Matriz Rotação ao Redor de Z Antihorária/1
  Constant2/1 -> Matriz Rotação ao Redor de Z Antihorária/2
  Constant3/1 -> Matriz Rotação ao Redor de Z Antihorária/3
  Constant4/1 -> Matriz Rotação ao Redor de Z Antihorária/4
  Trigonometric Function1/1 -> Matriz Rotação ao Redor de Z Antihorária/5
  Gain1/1 -> Matriz Rotação ao Redor de Z Antihorária/6
  Constant1/1 -> Matriz Rotação ao Redor de Z Antihorária/7
  Trigonometric Function2/1 -> Matriz Rotação ao Redor de Z Antihorária/8
  Trigonometric Function3/1 -> Matriz Rotação ao Redor de Z Antihorária/9
  Gain/1 -> Trigonometric Function1/1, Trigonometric Function/1, Trigonometric Function2/1, Trigonometric Function3/1

== system Simulacao_TCC_Final/Earth's Magnetic Field SGF/SGF para SGG2 ==
  B_SMG : Inport
  Constant{1..4} (4 alike) : Constant  Value=0
  Constant5 : Constant
  Constant6 : Constant  Value=11*(pi/180)
  Gain : Gain  Gain=-1
  Gain1 : Gain  Gain=-1
  Matriz Rotação ao Redor de Z Antihorária : sharedutil/Create 3x3 Matrix  aMode=aMode
  Trigonometric Function : Trigonometry
  Trigonometric Function1 : Trigonometry  Operator=cos
  Trigonometric Function2 : Trigonometry
  Trigonometric Function3 : Trigonometry  Operator=cos
  product 2 : Product  Multiplication=Matrix(*)  RndMeth=Zero
  B_SGG : Outport
  wires:
  Constant6/1 -> Gain/1
  product 2/1 -> B_SGG/1
  Trigonometric Function/1 -> Gain1/1
  Matriz Rotação ao Redor de Z Antihorária/1 -> product 2/1  "Matriz de Rotação"
  B_SMG/1 -> product 2/2
  Constant5/1 -> Matriz Rotação ao Redor de Z Antihorária/1
  Constant2/1 -> Matriz Rotação ao Redor de Z Antihorária/2
  Constant3/1 -> Matriz Rotação ao Redor de Z Antihorária/3
  Constant4/1 -> Matriz Rotação ao Redor de Z Antihorária/4
  Trigonometric Function1/1 -> Matriz Rotação ao Redor de Z Antihorária/5
  Gain1/1 -> Matriz Rotação ao Redor de Z Antihorária/6
  Constant1/1 -> Matriz Rotação ao Redor de Z Antihorária/7
  Trigonometric Function2/1 -> Matriz Rotação ao Redor de Z Antihorária/8
  Trigonometric Function3/1 -> Matriz Rotação ao Redor de Z Antihorária/9
  Gain/1 -> Trigonometric Function1/1, Trigonometric Function/1, Trigonometric Function2/1, Trigonometric Function3/1

== system Simulacao_TCC_Final/Earth's Magnetic Field SGF/SGF para SGG3 ==
  B_SGG : Inport
  Constant{1..4} (4 alike) : Constant  Value=0
  Constant5 : Constant
  Gain : Gain  Gain=-1
  Gain1 : Gain  Gain=-1
  Matriz Rotação ao Redor de Z Antihorária : sharedutil/Create 3x3 Matrix  aMode=aMode
  Rotação da Terra : simulink/Sources/Ramp  slope="7.292115856e-5   %2*pi/(24*60*60)  %radians/second (one rotation per day )"  start=0  InitialOutput=0
  Trigonometric Function : Trigonometry
  Trigonometric Function1 : Trigonometry  Operator=cos
  Trigonometric Function2 : Trigonometry
  Trigonometric Function3 : Trigonometry  Operator=cos
  product 2 : Product  Multiplication=Matrix(*)  RndMeth=Zero
  B_SGF : Outport
  wires:
  Rotação da Terra/1 -> Gain/1
  product 2/1 -> B_SGF/1
  Trigonometric Function1/1 -> Matriz Rotação ao Redor de Z Antihorária/1
  Trigonometric Function/1 -> Gain1/1
  Gain1/1 -> Matriz Rotação ao Redor de Z Antihorária/2
  Constant1/1 -> Matriz Rotação ao Redor de Z Antihorária/3
  Trigonometric Function2/1 -> Matriz Rotação ao Redor de Z Antihorária/4
  Trigonometric Function3/1 -> Matriz Rotação ao Redor de Z Antihorária/5
  Constant2/1 -> Matriz Rotação ao Redor de Z Antihorária/6
  Constant3/1 -> Matriz Rotação ao Redor de Z Antihorária/7
  Constant4/1 -> Matriz Rotação ao Redor de Z Antihorária/8
  Constant5/1 -> Matriz Rotação ao Redor de Z Antihorária/9
  Matriz Rotação ao Redor de Z Antihorária/1 -> product 2/1  "Matriz de Rotação"
  B_SGG/1 -> product 2/2
  Gain/1 -> Trigonometric Function2/1, Trigonometric Function3/1, Trigonometric Function/1, Trigonometric Function1/1

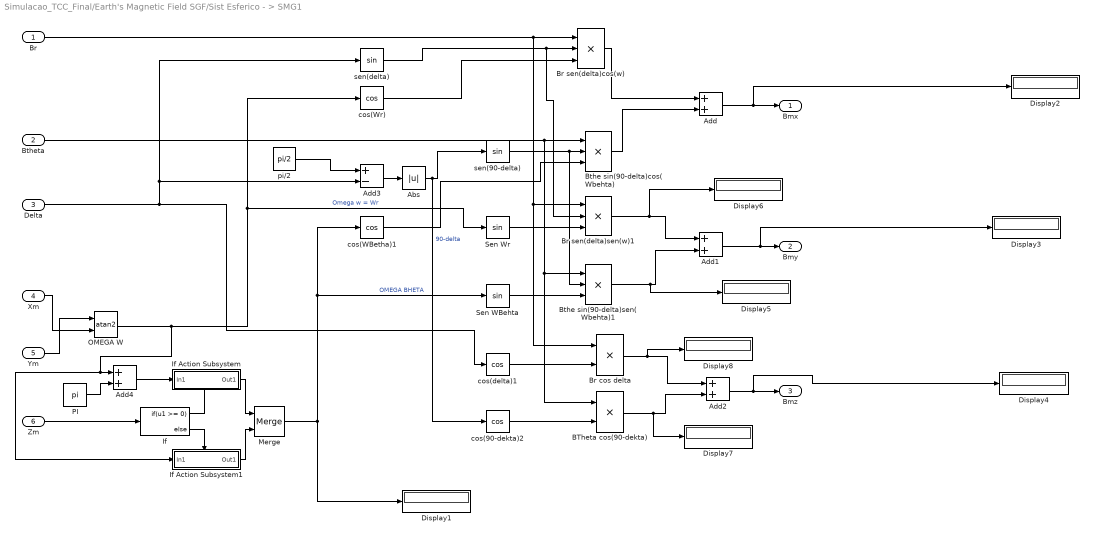
== system Simulacao_TCC_Final/Earth's Magnetic Field SGF/Sist Esferico - > SMG1 ==
  Br : Inport
  Btheta : Inport  Port=2
  Delta : Inport  Port=3
  Xm : Inport  Port=4
  Ym : Inport  Port=5
  Zm : Inport  Port=6
  Abs : Abs
  Add{,1..2,4} (4 alike) : Sum
  Add3 : Sum  Inputs=+-
  "BTheta cos(90-dekta) " : Product
  Br cos delta : Product
  Br sen(delta)cos(w) : Product  Inputs=3
  Br sen(delta)sen(w)1 : Product  Inputs=3
  Bthe sin(90-delta)cos(Wbehta) : Product  Inputs=3
  Bthe sin(90-delta)sen(Wbehta)1 : Product  Inputs=3
  Display{1..8} (8 alike) : Display
  If : If  IfExpression=u1 >= 0
  If Action Subsystem : Subsystem  TreatAsAtomicUnit=on
  If Action Subsystem1 : Subsystem  TreatAsAtomicUnit=on
  Merge : Merge
  OMEGA W : Trigonometry  Operator=atan2
  PI : Constant  Value=pi
  Sen WBehta : Trigonometry
  Sen Wr : Trigonometry
  cos(90-dekta)2 : Trigonometry  Operator=cos
  cos(WBetha)1 : Trigonometry  Operator=cos
  cos(Wr) : Trigonometry  Operator=cos
  cos(delta)1 : Trigonometry  Operator=cos
  "pi/2 " : Constant  Value=pi/2
  sen(90-delta) : Trigonometry
  sen(delta) : Trigonometry
  Bmx : Outport
  Bmy : Outport  Port=2
  Bmz : Outport  Port=3
  wires:
  Add1/1 -> Display3/1, Bmy/1
  Add/1 -> Display2/1, Bmx/1
  Ym/1 -> OMEGA W/1
  Xm/1 -> OMEGA W/2
  Br/1 -> Br cos delta/1, Br sen(delta)sen(w)1/1, Br sen(delta)cos(w)/1
  sen(delta)/1 -> Br sen(delta)sen(w)1/2, Br sen(delta)cos(w)/2
  Delta/1 -> cos(delta)1/1, sen(delta)/1, Add3/2
  cos(Wr)/1 -> Br sen(delta)cos(w)/3
  OMEGA W/1 -> If Action Subsystem1/1(In1), Add4/1, Sen Wr/1, cos(Wr)/1  "Omega w = Wr"
  Br sen(delta)cos(w)/1 -> Add/1
  Bthe sin(90-delta)cos(Wbehta)/1 -> Add/2
  Btheta/1 -> "BTheta cos(90-dekta) "/1, Bthe sin(90-delta)sen(Wbehta)1/1, Bthe sin(90-delta)cos(Wbehta)/1
  Add3/1 -> Abs/1
  Abs/1 -> cos(90-dekta)2/1, sen(90-delta)/1  "90-delta"
  "pi/2 "/1 -> Add3/1
  sen(90-delta)/1 -> Bthe sin(90-delta)cos(Wbehta)/2, Bthe sin(90-delta)sen(Wbehta)1/2
  If Action Subsystem/1(Out1) -> Merge/1
  If Action Subsystem1/1(Out1) -> Merge/2
  If/1 -> If Action Subsystem/Action
  If/2 -> If Action Subsystem1/Action
  Zm/1 -> If/1
  Add4/1 -> If Action Subsystem/1(In1)
  PI/1 -> Add4/2
  cos(WBetha)1/1 -> Bthe sin(90-delta)cos(Wbehta)/3
  Merge/1 -> Sen WBehta/1, cos(WBetha)1/1, Display1/1  "OMEGA BHETA"
  Sen Wr/1 -> Br sen(delta)sen(w)1/3
  Br sen(delta)sen(w)1/1 -> Display6/1, Add1/1
  Bthe sin(90-delta)sen(Wbehta)1/1 -> Display5/1, Add1/2
  Sen WBehta/1 -> Bthe sin(90-delta)sen(Wbehta)1/3
  "BTheta cos(90-dekta) "/1 -> Display7/1, Add2/2
  cos(delta)1/1 -> Br cos delta/2
  cos(90-dekta)2/1 -> "BTheta cos(90-dekta) "/2
  Add2/1 -> Display4/1, Bmz/1
  Br cos delta/1 -> Display8/1, Add2/1

== system Simulacao_TCC_Final/Eliptical Orbit/Calculo de E ==
  tempo : Inport
  Tal : Inport  Port=2
  T - periodo : Inport  Port=3
  "e  " : Inport  Port=4
  Calculo_E_Orbitas : MATLAB Function  TreatAsAtomicUnit=on
  Constant : Constant  Value=2
  Constant1 : Constant  Value=pi
  Display : Display
  Display1 : Display
  Divide : Product  Inputs=*/
  M : Product
  Mux1 : Mux  Inputs=2
  Product : Product
  Sum : Sum  Inputs=+-
  E : Outport
  wires:
  Constant/1 -> Product/1
  Constant1/1 -> Product/2
  Product/1 -> Divide/1
  T - periodo/1 -> Divide/2
  Divide/1 -> M/1
  Sum/1 -> M/2
  tempo/1 -> Sum/1
  Tal/1 -> Sum/2
  M/1 -> Display/1, Mux1/1  "M"
  "e  "/1 -> Display1/1, Mux1/2
  Mux1/1 -> Calculo_E_Orbitas/1(u)
  Calculo_E_Orbitas/1(E) -> E/1

== system Simulacao_TCC_Final/Eliptical Orbit/Calculo de Vr e V_thera ==
  e : Inport
  f : Inport  Port=2
  h : Inport  Port=3
  Add : Sum
  Constant : Constant
  Divide : Product  Inputs=*/
  Product : Product  Inputs=3
  Product1 : Product
  Product2 : Product
  Trigonometric Function : Trigonometry
  Trigonometric Function1 : Trigonometry  Operator=cos
  mi : Constant  Value=3.9886004418e14
  Vr : Outport
  V_theta : Outport  Port=2
  wires:
  Product/1 -> Vr/1
  Divide/1 -> Product1/1, Product/1
  mi/1 -> Divide/1
  h/1 -> Divide/2
  e/1 -> Product2/1, Product/2
  Trigonometric Function/1 -> Product/3
  f/1 -> Trigonometric Function1/1, Trigonometric Function/1
  Product1/1 -> V_theta/1
  Add/1 -> Product1/2
  Constant/1 -> Add/2
  Product2/1 -> Add/1
  Trigonometric Function1/1 -> Product2/2

== system Simulacao_TCC_Final/Eliptical Orbit/Calculo de f ==
  e : Inport
  E : Inport  Port=2
  1 : Constant
  Add : Sum
  Add1 : Sum  Inputs=+-
  Constant : Constant  Value=2
  Constant1 : Constant  Value=2
  Divide : Product  Inputs=*/
  Divide1 : Product  Inputs=*/
  Product : Product
  Product1 : Product
  Sqrt : Sqrt  SaturateOnIntegerOverflow=on
  Trigonometric Function : Trigonometry  Operator=atan
  Trigonometric Function1 : Trigonometry  Operator=tan
  f : Outport
  wires:
  Constant/1 -> Product/1
  Product/1 -> f/1
  Trigonometric Function/1 -> Product/2
  Product1/1 -> Trigonometric Function/1
  Sqrt/1 -> Product1/2
  Trigonometric Function1/1 -> Product1/1
  Divide/1 -> Trigonometric Function1/1
  Constant1/1 -> Divide/2
  E/1 -> Divide/1
  Add/1 -> Divide1/1
  Add1/1 -> Divide1/2
  Divide1/1 -> Sqrt/1
  1/1 -> Add1/1, Add/1
  e/1 -> Add1/2, Add/2

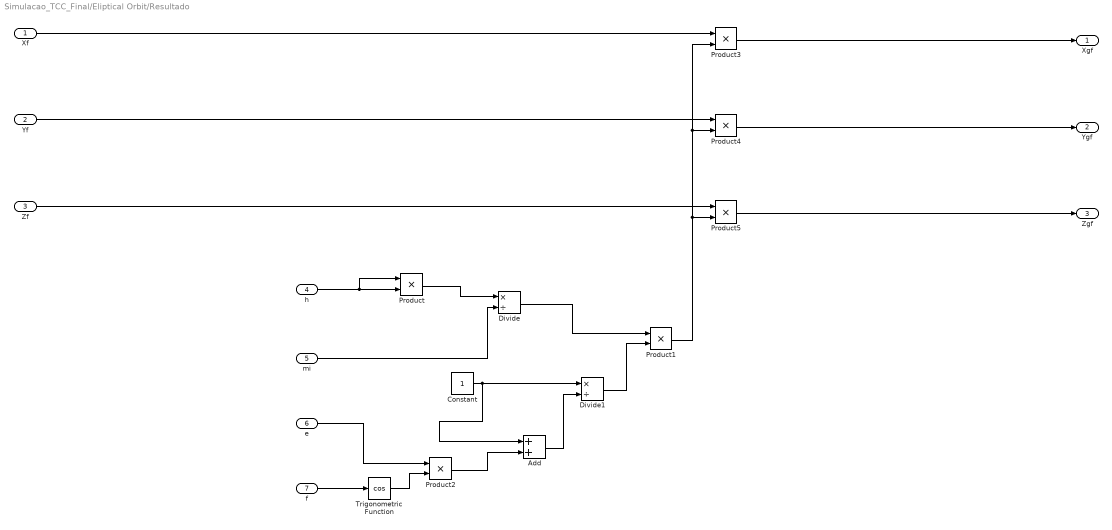
== system Simulacao_TCC_Final/Eliptical Orbit/Resultado ==
  Xf : Inport
  Yf : Inport  Port=2
  Zf : Inport  Port=3
  h : Inport  Port=4
  mi : Inport  Port=5
  e : Inport  Port=6
  f : Inport  Port=7
  Add : Sum
  Constant : Constant
  Divide : Product  Inputs=*/
  Divide1 : Product  Inputs=*/
  Product{,1..5} (6 alike) : Product
  Trigonometric Function : Trigonometry  Operator=cos
  Xgf : Outport
  Ygf : Outport  Port=2
  Zgf : Outport  Port=3
  wires:
  h/1 -> Product/2, Product/1
  mi/1 -> Divide/2
  Product/1 -> Divide/1
  Divide/1 -> Product1/1
  Constant/1 -> Add/1, Divide1/1
  e/1 -> Product2/1
  f/1 -> Trigonometric Function/1
  Trigonometric Function/1 -> Product2/2
  Product2/1 -> Add/2
  Add/1 -> Divide1/2
  Divide1/1 -> Product1/2
  Xf/1 -> Product3/1
  Yf/1 -> Product4/1
  Zf/1 -> Product5/1
  Product1/1 -> Product5/2, Product4/2, Product3/2
  Product3/1 -> Xgf/1
  Product4/1 -> Ygf/1
  Product5/1 -> Zgf/1

== system Simulacao_TCC_Final/Eliptical Orbit/T - Periodo ==
  a : Inport
  Constant : Constant  Value=2
  Divide : Product  Inputs=*/
  PI : Constant  Value=pi
  Product : Product
  Product1 : Product
  Product2 : Product  Inputs=3
  Sqrt : Sqrt  SaturateOnIntegerOverflow=on
  mi - metros : Constant  Value=3.9886004418e14
  T : Outport
  wires:
  Product/1 -> T/1
  Product1/1 -> Product/1
  PI/1 -> Product1/2
  Constant/1 -> Product1/1
  Sqrt/1 -> Product/2
  Divide/1 -> Sqrt/1
  mi - metros/1 -> Divide/2
  a/1 -> Product2/1, Product2/3, Product2/2
  Product2/1 -> Divide/1

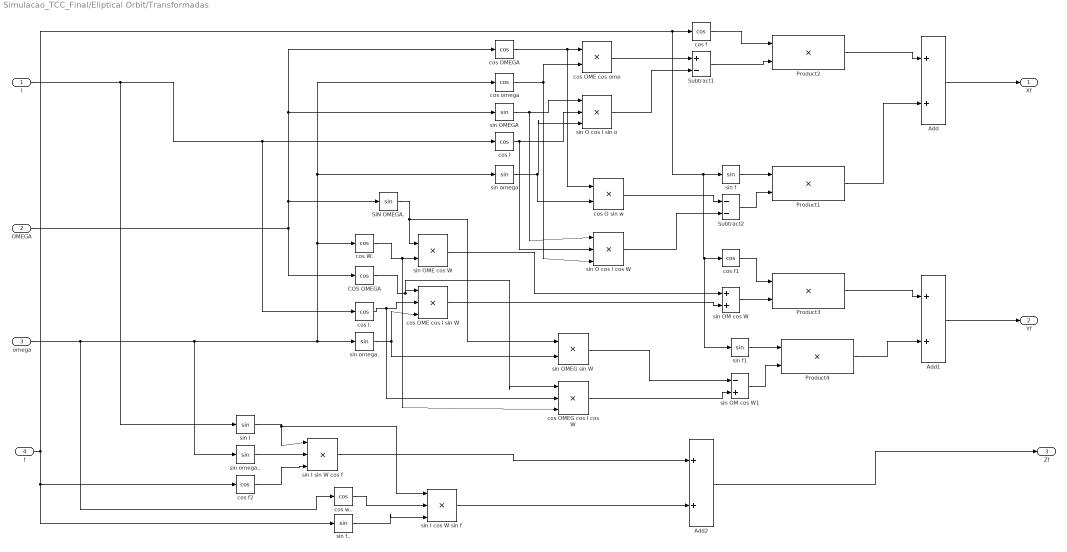
== system Simulacao_TCC_Final/Eliptical Orbit/Transformadas ==
  I : Inport
  OMEGA : Inport  Port=2
  omega : Inport  Port=3
  f : Inport  Port=4
  Add : Sum
  Add1 : Sum
  Add2 : Sum
  COS OMEGA : Trigonometry  Operator=cos
  Product{1..4} (4 alike) : Product
  SIN OMEGA. : Trigonometry
  Subtract1 : Sum  Inputs=+-
  Subtract2 : Sum  Inputs=--
  cos I : Trigonometry  Operator=cos
  cos I. : Trigonometry  Operator=cos
  cos O sin w : Product
  cos OME cos I sin W : Product  Inputs=3
  cos OME cos ome : Product
  cos OMEG cos I cos W : Product  Inputs=3
  cos OMEGA : Trigonometry  Operator=cos
  cos W. : Trigonometry  Operator=cos
  cos f : Trigonometry  Operator=cos
  cos f1 : Trigonometry  Operator=cos
  cos f2 : Trigonometry  Operator=cos
  cos omega : Trigonometry  Operator=cos
  cos w.. : Trigonometry  Operator=cos
  sin I : Trigonometry
  sin I cos W sin f : Product  Inputs=3
  sin I sin W cos f : Product  Inputs=3
  sin O cos I cos W : Product  Inputs=3
  sin O cos I sin o : Product  Inputs=3
  sin OM cos W : Sum
  sin OM cos W1 : Sum  Inputs=-+
  sin OME cos W : Product
  sin OMEG sin W : Product
  sin OMEGA : Trigonometry
  sin f : Trigonometry
  sin f.. : Trigonometry
  sin f1 : Trigonometry
  sin omega : Trigonometry
  "sin omega. " : Trigonometry
  sin omega.. : Trigonometry
  Xf : Outport
  Yf : Outport  Port=2
  Zf : Outport  Port=3
  wires:
  Add/1 -> Xf/1
  Add1/1 -> Yf/1
  Add2/1 -> Zf/1
  Product2/1 -> Add/1
  Product1/1 -> Add/2
  Subtract1/1 -> Product2/2
  cos f/1 -> Product2/1
  cos OME cos ome/1 -> Subtract1/1
  sin O cos I sin o/1 -> Subtract1/2
  OMEGA/1 -> SIN OMEGA./1, sin OMEGA/1, cos OMEGA/1, COS OMEGA/1
  cos OMEGA/1 -> cos O sin w/1, cos OME cos ome/1
  omega/1 -> cos w../1, sin omega../1, cos W./1, cos omega/1, sin omega/1, "sin omega. "/1
  cos I/1 -> sin O cos I cos W/2, sin O cos I sin o/2
  I/1 -> sin I/1, cos I./1, cos I/1
  f/1 -> sin f../1, cos f2/1, sin f1/1, cos f1/1, sin f/1, cos f/1
  Subtract2/1 -> Product1/2
  sin f/1 -> Product1/1
  cos O sin w/1 -> Subtract2/1
  sin O cos I cos W/1 -> Subtract2/2
  sin omega/1 -> cos O sin w/2, sin O cos I sin o/3
  sin OMEGA/1 -> sin O cos I cos W/1, sin O cos I sin o/1
  cos omega/1 -> sin O cos I cos W/3, cos OME cos ome/2
  Product3/1 -> Add1/1
  Product4/1 -> Add1/2
  cos f1/1 -> Product3/1
  sin OM cos W/1 -> Product3/2
  sin OME cos W/1 -> sin OM cos W/1
  cos OME cos I sin W/1 -> sin OM cos W/2
  cos W./1 -> cos OMEG cos I cos W/3, sin OME cos W/2
  COS OMEGA/1 -> cos OMEG cos I cos W/1, cos OME cos I sin W/1
  cos I./1 -> cos OMEG cos I cos W/2, cos OME cos I sin W/2
  "sin omega. "/1 -> cos OME cos I sin W/3, sin OMEG sin W/2
  sin f1/1 -> Product4/1
  sin OM cos W1/1 -> Product4/2
  sin OMEG sin W/1 -> sin OM cos W1/1
  cos OMEG cos I cos W/1 -> sin OM cos W1/2
  SIN OMEGA./1 -> sin OMEG sin W/1, sin OME cos W/1
  sin I sin W cos f/1 -> Add2/1
  sin I cos W sin f/1 -> Add2/2
  sin I/1 -> sin I cos W sin f/1, sin I sin W cos f/1
  sin omega../1 -> sin I sin W cos f/2
  cos f2/1 -> sin I sin W cos f/3
  cos w../1 -> sin I cos W sin f/2
  sin f../1 -> sin I cos W sin f/3

== system Simulacao_TCC_Final/Eliptical Orbit/h - Momento Angular da Orbita ==
  e : Inport
  a : Inport  Port=2
  1 : Constant
  Add : Sum  Inputs=+-
  Math Function : Math  Operator=magnitude^2  SaturateOnIntegerOverflow=on
  Product : Product  Inputs=3
  Sqrt : Sqrt  SaturateOnIntegerOverflow=on
  mi - metros : Constant  Value=3.9886004418e14
  h : Outport
  wires:
  Sqrt/1 -> h/1
  Product/1 -> Sqrt/1
  a/1 -> Product/1
  mi - metros/1 -> Product/2
  Add/1 -> Product/3
  1/1 -> Add/1
  Math Function/1 -> Add/2
  e/1 -> Math Function/1

== system Simulacao_TCC_Final/Gradient Gravity Torque/Calculo da Posição no Corpo ==
  X_SGF : Inport
  Euler : Inport  Port=2
  Demux1 : Demux  Outputs=3
  Matrix Multiply : Product  Multiplication=Matrix(*)
  Matrix Multiply1 : Product  Multiplication=Matrix(*)
  Matrix Multiply2 : Product  Multiplication=Matrix(*)
  Matrix de Rotação em X : Subsystem
  Matrix de Rotação em Y : Subsystem
  Matrix de Rotação em Z : Subsystem
  X_SCS : Outport
  wires:
  X_SGF/1 -> Matrix Multiply/2
  Matrix Multiply/1 -> X_SCS/1
  Matrix de Rotação em X/1(Matrix Rotação  em X) -> Matrix Multiply1/1
  Euler/1 -> Demux1/1
  Demux1/3 -> Matrix de Rotação em Z/1(Phi)
  Matrix de Rotação em Z/1(Matrix Rotação  em Z) -> Matrix Multiply2/2
  Matrix de Rotação em Y/1(Matrix Rotação  em Y) -> Matrix Multiply1/2
  Demux1/2 -> Matrix de Rotação em Y/1(Gamma)
  Matrix Multiply1/1 -> Matrix Multiply2/1
  Matrix Multiply2/1 -> Matrix Multiply/1
  Demux1/1 -> Matrix de Rotação em X/1(Phi)

== system Simulacao_TCC_Final/Hysteresis Torque/Hysteresys ==
  H : Inport
  Constant1 : Constant  Value=0.73* (1e4)
  Constant2 : Constant  Value=0.35* (1e4)
  Constant3 : Constant  Value=1.59
  Derivative : Derivative
  Gain : Gain  Gain=10000
  Gain2 : Gain  Gain=1/10000
  Hysteresis Loop : MATLAB Function  TreatAsAtomicUnit=on
  Integrator : Integrator  InitialCondition=10000
  Rate Transition : RateTransition  Deterministic=off  OutPortSampleTimeOpt=Inherit  OutPortSampleTime=0.05
  Saturation1 : Saturate  UpperLimit=0.73  LowerLimit=-0.73
  B : Outport
  wires:
  Hysteresis Loop/1(DB_DT) -> Integrator/1
  Integrator/1 -> Gain2/1
  Gain/1 -> Hysteresis Loop/1(B)
  Gain2/1 -> Saturation1/1
  Saturation1/1 -> Gain/1, B/1
  Rate Transition/1 -> Hysteresis Loop/2(H), Derivative/1
  Derivative/1 -> Hysteresis Loop/3(DHDT)
  H/1 -> Rate Transition/1
  Constant1/1 -> Hysteresis Loop/4(Bs)
  Constant2/1 -> Hysteresis Loop/5(Br)
  Constant3/1 -> Hysteresis Loop/6(Hc)

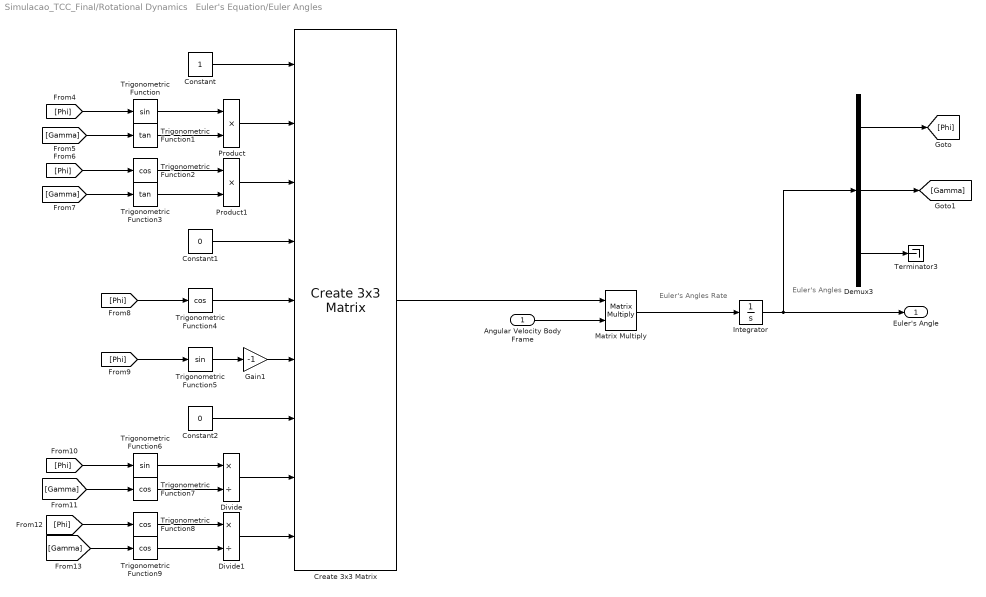
== system Simulacao_TCC_Final/Rotational Dynamics   Euler's Equation/Euler Angles ==
  note: Euler's Angles
  note: Euler's Angles
      | Rate
  Angular Velocity Body Frame : Inport
  Constant : Constant
  Constant1 : Constant  Value=0
  Constant2 : Constant  Value=0
  Create 3x3 Matrix : sharedutil/Create 3x3 Matrix  aMode=aMode
  Demux3 : Demux  Outputs=3
  Divide : Product  Inputs=*/
  Divide1 : Product  Inputs=*/
  Gain1 : Gain  Gain=-1
  Integrator : Integrator
  Matrix Multiply : Product  Multiplication=Matrix(*)
  Product : Product
  Product1 : Product
  Terminator3 : Terminator
  Trigonometric Function : Trigonometry
  Trigonometric Function1 : Trigonometry  Operator=tan
  Trigonometric Function{2,4,7..9} (5 alike) : Trigonometry  Operator=cos
  Trigonometric Function3 : Trigonometry  Operator=tan
  Trigonometric Function5 : Trigonometry
  Trigonometric Function6 : Trigonometry
  Euler's Angle : Outport
  wires:
  Create 3x3 Matrix/1 -> Matrix Multiply/1
  Angular Velocity Body Frame/1 -> Matrix Multiply/2
  Matrix Multiply/1 -> Integrator/1
  Constant/1 -> Create 3x3 Matrix/1
  Product/1 -> Create 3x3 Matrix/2
  Trigonometric Function/1 -> Product/1
  Trigonometric Function1/1 -> Product/2
  [Phi] -> Trigonometric Function/1
  [Gamma] -> Trigonometric Function1/1
  [Phi] -> Trigonometric Function2/1
  [Gamma] -> Trigonometric Function3/1
  Product1/1 -> Create 3x3 Matrix/3
  Trigonometric Function2/1 -> Product1/1
  Trigonometric Function3/1 -> Product1/2
  Constant1/1 -> Create 3x3 Matrix/4
  Trigonometric Function4/1 -> Create 3x3 Matrix/5
  [Phi] -> Trigonometric Function4/1
  [Phi] -> Trigonometric Function5/1
  Trigonometric Function5/1 -> Gain1/1
  Gain1/1 -> Create 3x3 Matrix/6
  Constant2/1 -> Create 3x3 Matrix/7
  Divide/1 -> Create 3x3 Matrix/8
  Divide1/1 -> Create 3x3 Matrix/9
  [Phi] -> Trigonometric Function6/1
  [Gamma] -> Trigonometric Function7/1
  Trigonometric Function6/1 -> Divide/1
  Trigonometric Function7/1 -> Divide/2
  Trigonometric Function8/1 -> Divide1/1
  [Gamma] -> Trigonometric Function9/1
  [Phi] -> Trigonometric Function8/1
  Trigonometric Function9/1 -> Divide1/2
  Integrator/1 -> Euler's Angle/1, Demux3/1
  Demux3/1 -> [Phi]
  Demux3/2 -> [Gamma]
  Demux3/3 -> Terminator3/1

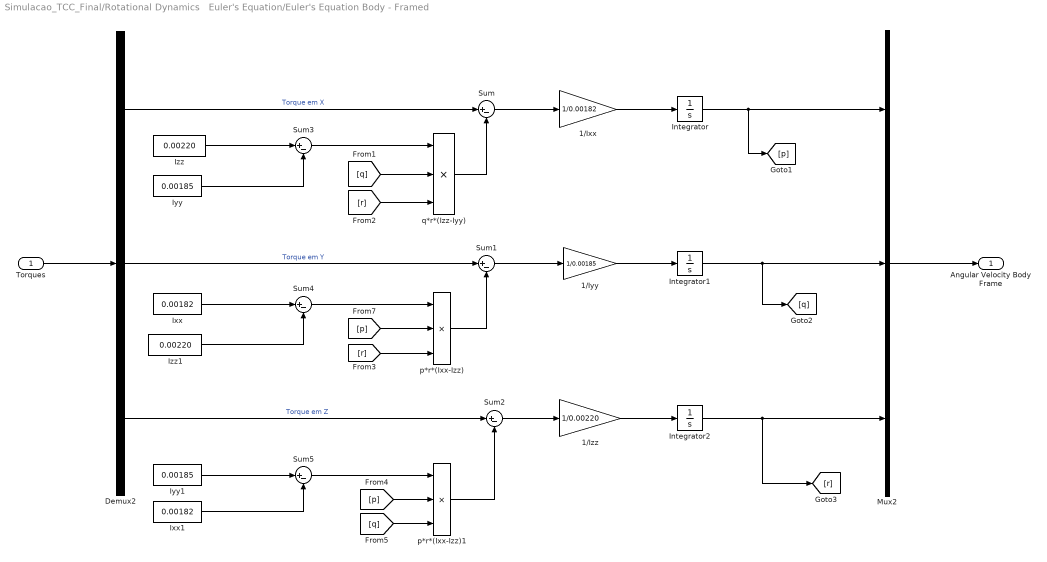
== system Simulacao_TCC_Final/Rotational Dynamics   Euler's Equation/Euler's Equation Body - Framed ==
  Torques : Inport
  1/Ixx : Gain  Gain=1/0.00182
  1/Iyy : Gain  Gain=1/0.00185
  1/Izz : Gain  Gain=1/0.00220
  Demux2 : Demux  Outputs=3
  Integrator : Integrator  InitialCondition=0.1
  Integrator1 : Integrator  InitialCondition=0.052
  Integrator2 : Integrator  InitialCondition=0.069
  Ixx : Constant  Value=0.00182
  Ixx1 : Constant  Value=0.00182
  Iyy : Constant  Value=0.00185
  Iyy1 : Constant  Value=0.00185
  Izz : Constant  Value=0.00220
  Izz1 : Constant  Value=0.00220
  Mux2 : Mux  Inputs=3
  Sum{,1..5} (6 alike) : Sum  Inputs=|+-
  p*r*(Ixx-Izz) : Product  Inputs=3
  p*r*(Ixx-Izz)1 : Product  Inputs=3
  q*r*(Izz-Iyy) : Product  Inputs=3
  Angular Velocity Body Frame : Outport
  wires:
  Integrator/1 -> Mux2/1, [p]
  Integrator1/1 -> Mux2/2, [q]
  Integrator2/1 -> Mux2/3, [r]
  1/Ixx/1 -> Integrator/1
  1/Iyy/1 -> Integrator1/1
  1/Izz/1 -> Integrator2/1
  Sum1/1 -> 1/Iyy/1
  Sum/1 -> 1/Ixx/1
  Sum2/1 -> 1/Izz/1
  Torques/1 -> Demux2/1
  Demux2/1 -> Sum/1  "Torque em X"
  Demux2/2 -> Sum1/1  "Torque em Y"
  Demux2/3 -> Sum2/1  "Torque em Z"
  q*r*(Izz-Iyy)/1 -> Sum/2
  p*r*(Ixx-Izz)/1 -> Sum1/2
  p*r*(Ixx-Izz)1/1 -> Sum2/2
  Sum3/1 -> q*r*(Izz-Iyy)/1
  Izz/1 -> Sum3/1
  Iyy/1 -> Sum3/2
  [q] -> q*r*(Izz-Iyy)/2
  [r] -> q*r*(Izz-Iyy)/3
  Sum4/1 -> p*r*(Ixx-Izz)/1
  Izz1/1 -> Sum4/2
  Ixx/1 -> Sum4/1
  [p] -> p*r*(Ixx-Izz)/2
  [r] -> p*r*(Ixx-Izz)/3
  Sum5/1 -> p*r*(Ixx-Izz)1/1
  Ixx1/1 -> Sum5/2
  Iyy1/1 -> Sum5/1
  [p] -> p*r*(Ixx-Izz)1/2
  [q] -> p*r*(Ixx-Izz)1/3
  Mux2/1 -> Angular Velocity Body Frame/1
